simulink model "Problem2_Linearized"  (R2018a)
settings: Solver=VariableStepAuto  StartTime=0.0  StopTime=tStop  MaxStep=T/4  RelTol=1e-3
values from neighbouring files (symbols this model uses):
  A2 = [-D*Ron/L -(1-D)/(n*L); (1-D)/(n*C) -1/(R*C)]    [EE458_HW1_Solution.m]
  B2 = [(Vg - I2*Ron + V2/n)/L D/L; -I2/(n*C) 0]    [EE458_HW1_Solution.m]
  d_after = 0.75    [EE458_HW1_Solution.m]
  d_before = 0.5    [EE458_HW1_Solution.m]
  tStepDuty = 40e-3    (= 0.04)    [EE458_HW1_Solution.m]
  tStepVg = 20e-3    (= 0.02)    [EE458_HW1_Solution.m]
  U = [D; Vg]    [EE458_HW1_Solution.m]
  vg_after = 75    [EE458_HW1_Solution.m]
  vg_before = 100    [EE458_HW1_Solution.m]
  X2 = n*D*Vg*[n; (1-D)*R]/(D*n^2*Ron + R*(1 - D)^2)    [EE458_HW1_Solution.m]
settings Model: Creator=brianbj  LastModifiedBy=brianbj

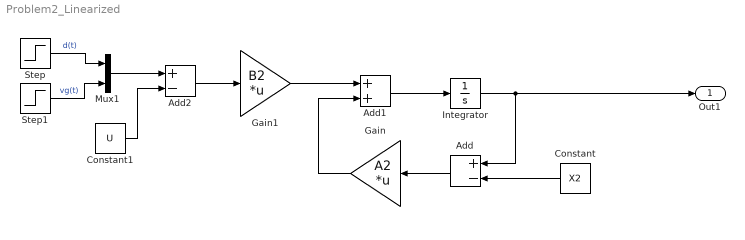
== system Problem2_Linearized ==
  Add : Sum  Inputs=+-
  Add1 : Sum
  Add2 : Sum  Inputs=+-
  Constant : Constant  Value=X2
  Constant1 : Constant  Value=U
  Gain : Gain  Gain=A2  Multiplication=Matrix(K*u) (u vector)
  Gain1 : Gain  Gain=B2  Multiplication=Matrix(K*u) (u vector)
  Integrator : Integrator  InitialCondition=X2
  Mux1 : Mux  Inputs=2
  Step : Step  Time=tStepDuty  Before=d_before  After=d_after  SampleTime=0
  Step1 : Step  Time=tStepVg  Before=vg_before  After=vg_after  SampleTime=0
  Out1 : Outport
  wires:
  Integrator/1 -> Out1/1, Add/1
  Add/1 -> Gain/1
  Add1/1 -> Integrator/1
  Gain1/1 -> Add1/1
  Gain/1 -> Add1/2
  Add2/1 -> Gain1/1
  Constant/1 -> Add/2
  Constant1/1 -> Add2/2
  Step1/1 -> Mux1/2  "vg(t)"
  Step/1 -> Mux1/1  "d(t)"
  Mux1/1 -> Add2/1
